simulink library "vxlib1"  (Simulink 6.0)
settings: Solver=ode45  SolverMode=SingleTasking  StartTime=0.0  StopTime=10.0  RelTol=1e-3
settings Model: Creator=jwu  LastModifiedBy=jcarrick  ExtModeAutoUpdateStatusClock=off
settings DataIOCC: SignalLoggingName=logsOut
settings OptimizationCC: BooleanDataType=off
settings DebuggingCC: CheckExecutionContextPreStartOutputMsg=on  CheckExecutionContextRuntimeOutputMsg=on  SolverPrmCheckMsg=none
settings HardwareCC: TargetUnknown=on
settings SFSimCC: SFSimApplyToAllLibs=on  SFSimBuildMode=Incremental

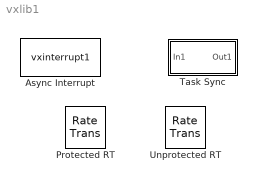
== system vxlib1 ==
  Async Interrupt : S-Function  FunctionName=vxinterrupt1  Parameters=irqnumbers, irqoffsets, irqpriorities, irqpreempts, showinput,tickres  mask(VxWorks Interrrupt Block){irqnumbers=[1 2], irqoffsets=[192 193], irqpriorities=[10 11], irqpreempts=[0 1], tickres=1/60, showinput=on}
      mask prompts: irqnumbers "VME interrupt number(s):"; irqoffsets "VME interrupt vector offset(s):"; irqpriorities "Effective priority(s):"; irqpreempts "Preemption flag(s): preemptable-1, non-preemptable-0"; tickres "Timer resolution (seconds):"; showinput "Enable simulation input:"
      mask help: Create VME based Interrupt Service Routine which will execute the downstream subsystem or Task Block.
      mask init:
      | devicedir = fullfile(matlabroot,'rtw','c','tornado','devices');
      | if isempty(findstr(devicedir, path))
      | 	addpath(devicedir);
      | end
      | 
      | irqstr = num2str(irqnumbers);
      | if length(irqstr) ~= 1
      | 	irqstr = 'N';
      | end
      | 
      | if ~showinput
      | 	% make the input port label disappear
      | 	pvalue = irqstr;
      | 	pname = 'output';
      | else
      | 	pvalue = 'SimIRQ';
      | 	pname = 'input';
      | end
      | if strcmp(get_param(bdroot(gcbh),'BlockDiagramType'),'model')
      |   cs = getActiveConfigSet(bdroot);
      |   if strcmp(get_param(cs, 'SampleTimeConstraint'), 'Specified')
      |     stprop = get_param(cs, 'SampleTimeProperty');
      |     basepriority = stprop(1).Priority;
      |   else
      |     % Simulink default is 40
      |     basepriority = 40;
      |   end
      |   intpris = get_param(gcb,'MaskValues');
      |   pri = eval(intpris{3});
      |   for i=1:length(pri)
      |     if pri(i)>= basepriority
      |       errTxt = ['Interrupt Block ''', gcb, ''' specifies a priority of ''',num2str(pri(i)), ...
      |                 ''' which is lower priority (higher value) or the same as the periodic ', ...
      |                 'base rate priority of ''',num2str(basepriority), '''. Please specify ',...
      |                 'a smaller ''Effective priority'' value.'];
      |       errordlg(errTxt,'Interrupt Priority Error','modal');
      |     end
      |   end
      | end
      mask Help: helpview([docroot '/mapfiles/rtw_ug.map'], 'rtw_async_support');
      mask Display:
      | port_label('output',1,['IRQ' irqstr])
      | port_label(pname,1,pvalue)
  Protected RT : RateTransition  Deterministic=off
  Task Sync : Subsystem  PropExecContextAcrossSSBoundary=on  mask(VxWorks Task Block){taskname=Task0, taskpriority=50, taskstacksize=8192, parentmanaget=off, tickres=1/60}
      mask prompts: taskname "Task name (10 characters or less):"; taskpriority "Task priority (0-255):"; taskstacksize "Stack size (bytes):"; parentmanaget "Synchronize the data transfer of this task with the caller task"; tickres "Timer resolution (seconds)"
      mask help: Creates a Task function which is spawned as a separate VxWorks Task. The Task function runs the code of the downstream function-call subsystem. When this block is run, a semaphore is used to enable the task execution.
      mask init:
      | devicedir = fullfile(matlabroot,'rtw','c','tornado','devices');
      | if isempty(findstr(devicedir, path))
      | 	addpath(devicedir);
      | end
      | 
      | if ~iscvar(taskname)
      |    errordlg('invalid Task Name, first character must be a letter or underscore and remaining characters must be letters,underscores or numbers.','Task Block Error','replace');
      |    taskname = '';
      | end
      mask Help: helpview([docroot '/mapfiles/rtw_ug.map'], 'rtw_async_support');
      mask CallbackString: |||a=get_param(gcb,'MaskValues');if strcmp(a{4},'on'), set_param(gcb,'MaskVisibilities',{'on','on','on','on','off'});else,set_param(gcb,'MaskVisibilities',{'on','on','on','on','on'});end|
      mask Display: disp(['Task\n''',taskname,''''])
  Unprotected RT : RateTransition  Integrity=off

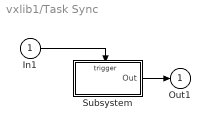
== system vxlib1/Task Sync ==
  In1 : Inport  LatchInput=off
  Subsystem : Subsystem  TreatAsAtomicUnit=on  PropExecContextAcrossSSBoundary=on
      settings: RTWSystemCode=Inline
      mask Type: VxWorks Task Block
  Out1 : Outport
  wires:
  Subsystem/1(Out) -> Out1/1
  In1/1 -> Subsystem/Trigger

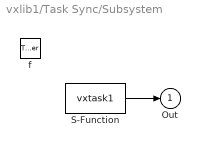
== system vxlib1/Task Sync/Subsystem ==
  f : TriggerPort  TriggerType=function-call
  S-Function : S-Function  FunctionName=vxtask1  Parameters=taskname, taskpriority, taskstacksize, parentmanaget, tickres
  Out : Outport
  wires:
  S-Function/1 -> Out/1
